simulink model "aero421_finalProjectSim_Part5"  (R2024a)
settings: Solver=FixedStepAuto  StartTime=0.0  StopTime=3*Period  FixedStep=10  RelTol=1e-3
values from neighbouring files (symbols this model uses):
  Kd = 0.6116*diag(3)    [aero421_finalProject.m]    (also in aero421_finalProject_D.m = 2*zeta*wn*detumbSat.Jrw)
  Kp = 7.035e-4*diag(3)    [aero421_finalProject.m]    (also in aero421_finalProject_D.m = wn^2*detumbSat.Jrw)
  q0 = [n0;e0]    [aero421_finalProject.m]    (also in aero421_finalProject_D.m)
undefined symbols (not defined in the file or in its folder): detumbSat
settings Model: Creator=emehiel  LastModifiedBy=joels
settings SolverCC: AlgebraicLoopSolver=TrustRegion
settings DebuggingCC: UnconnectedInputMsg=warning  UnconnectedOutputMsg=warning  UnconnectedLineMsg=warning
settings ModelReferenceCC: EnableRefExpFcnMdlSchedulingChecks=on
settings RTWCC: GPUComputeCapability=3.5

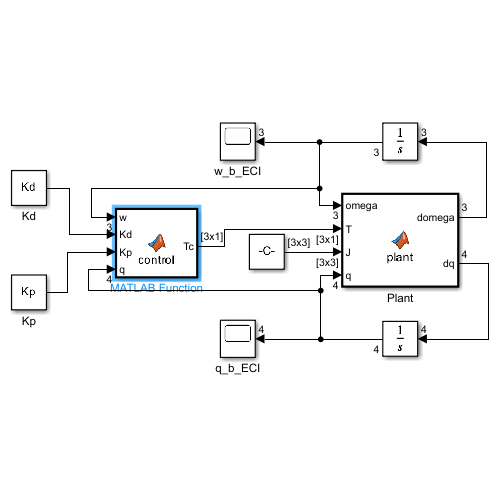
[thumbnail: Simulink's stored preview of the top-level diagram]
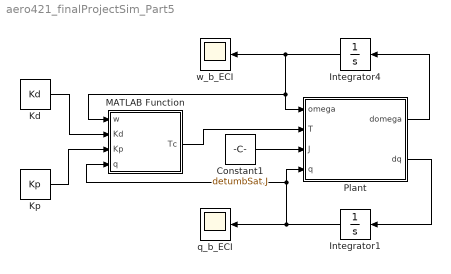
== system aero421_finalProjectSim_Part5 ==
  Constant1 : Constant  Value=detumbSat.J
  Integrator1 : Integrator  InitialCondition=q0
  Integrator4 : Integrator  InitialCondition=detumbSat.w0
  Kd : Constant  Value=Kd
  Kp : Constant  Value=Kp
  MATLAB Function : MATLAB Function  TreatAsAtomicUnit=on
  Plant : MATLAB Function  TreatAsAtomicUnit=on
  q_b_ECI : Scope
  w_b_ECI : Scope
  wires:
  Constant1/1 -> Plant/3(J)
  Plant/1(domega) -> Integrator4/1
  Integrator4/1 -> w_b_ECI/1, Plant/1(omega), MATLAB Function/1(w)
  Plant/2(dq) -> Integrator1/1
  Integrator1/1 -> q_b_ECI/1, Plant/4(q), MATLAB Function/4(q)
  Kp/1 -> MATLAB Function/3(Kp)
  Kd/1 -> MATLAB Function/2(Kd)
  MATLAB Function/1(Tc) -> Plant/2(T)

== matlab function aero421_finalProjectSim_Part5/MATLAB Function ==
  data: w input; Kd input; Kp input; q input; Tc output
function Tc = control(w,Kd,Kp,q)

% edot = w/2

qc = [-1;0;0;0];

qe = quatMult(qc,q);

epsilonError = qe(2:4);

Tc = -Kp*epsilonError - Kd*w;

% A = [zeros(3,3),eye(3);-1/2*inverse(I)*Kp,-inverse(I)*Kd];
% 
% xDot = A * [e,edot];

function qAns = quatMult(q1,q2)
% Quaternion Multiplication
% Inputs: Two quaternions in form [n;e]

w1 = q1(1);
x1 = q1(2);
y1 = q1(3);
z1 = q1(4);

w2 = q2(1);
x2 = q2(2);
y2 = q2(3);
z2 = q2(4);

qAns = [(w1*w2 - x1*x2 - y1*y2 - z1*z2); ...
        (w1*x2 + x1*w2 + y1*z2 - z1*y2); ...
        (w1*y2 - x1*z2 + y1*w2 + z1*x2); ...
        (w1*z2 + x1*y2 - y1*x2 + z1*w2)];
end
end

== matlab function aero421_finalProjectSim_Part5/Plant ==
  data: domega output; dq output; omega input; T input; J input; q input
function [domega,dq] = plant(omega, T, J, q)
%#codegen

norm(q)

% Compute the derivative of the angular velocity $\omega$ here

% Using the Euler Equations and T = 0

wXdot = (T(1)-(J(3,3)-J(2,2))*omega(2)*omega(3))/J(1,1);
wYdot = (T(2)-(J(1,1)-J(3,3))*omega(1)*omega(3))/J(2,2);
wZdot = (T(3)-(J(2,2)-J(1,1))*omega(1)*omega(2))/J(3,3);
domega = [wXdot; wYdot; wZdot];

n = q(1);
e = q(2:4);

dn = -1/2 * e' * omega;
de =  1/2 * ((n * eye(3)) + vect2cross(e)) * omega;

dq = [dn; de];
